simulink model "MBK"  (R2024a)
settings: Solver=ode4  StartTime=0.0  StopTime=20  FixedStep=0.01  RelTol=1e-3
InitFcn:
  | %% Initial Condition
  | m = 10;
  | b = 2;
  | k = 5;
settings Model: Creator=Ali  LastModifiedBy=Ali
settings SolverCC: AlgebraicLoopSolver=TrustRegion
settings DataIOCC: ReturnWorkspaceOutputs=off
settings DebuggingCC: UnconnectedInputMsg=warning  UnconnectedOutputMsg=warning  UnconnectedLineMsg=warning  ArithmeticOperatorsInVariantConditions=warning
settings ModelReferenceCC: EnableRefExpFcnMdlSchedulingChecks=on
settings SFSimCC: SimUseLocalCustomCode=off  CustomCodeUndefinedFunction=UseInterfaceOnly
settings RTWCC: RTWUseLocalCustomCode=off  GPUComputeCapability=3.5

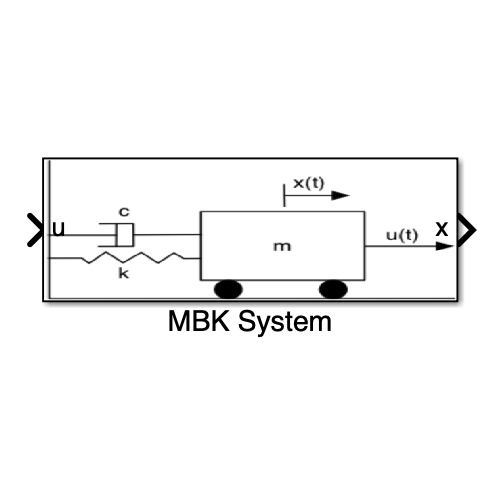
[thumbnail: Simulink's stored preview of the top-level diagram]
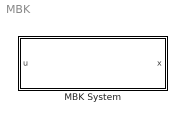
== system MBK ==
  MBK System : Subsystem
      mask Display: image('MBKPic.png');

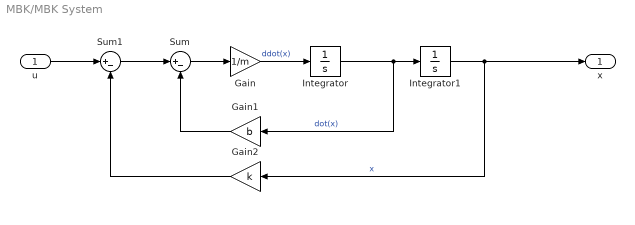
== system MBK/MBK System ==
  u : Inport
  Gain : Gain  Gain=1/m
  Gain1 : Gain  Gain=b
  Gain2 : Gain  Gain=k
  Integrator : Integrator
  Integrator1 : Integrator  InitialCondition=-1.519
  Sum : Sum  Inputs=|+-
  Sum1 : Sum  Inputs=|+-
  x : Outport
  wires:
  Gain2/1 -> Sum1/2
  Gain/1 -> Integrator/1  "ddot(x)"
  Integrator/1 -> Gain1/1, Integrator1/1  "dot(x)"
  u/1 -> Sum1/1
  Sum/1 -> Gain/1
  Gain1/1 -> Sum/2
  Integrator1/1 -> x/1, Gain2/1  "x"
  Sum1/1 -> Sum/1
